simulink library "Wheels_Driver_VehDyn_Lib"  (R2018a)
settings: Solver=VariableStepAuto  StartTime=0.0  StopTime=10.0  RelTol=1e-3
undefined symbols (not defined in the file): I, Kbr, P, vehicleMass
libraries: autolibshared x3, simulink x1
(part 3 of 3)

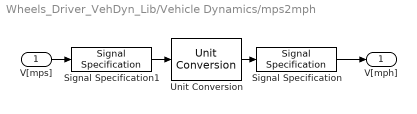
== system Wheels_Driver_VehDyn_Lib/Vehicle Dynamics/mps2mph ==
  V[mps] : Inport
  Signal Specification : SignalSpecification  Unit=mph
  Signal Specification1 : SignalSpecification  Unit=m/s
  Unit Conversion : UnitConversion
  V[mph] : Outport
  wires:
  V[mps]/1 -> Signal Specification1/1
  Unit Conversion/1 -> Signal Specification/1
  Signal Specification1/1 -> Unit Conversion/1
  Signal Specification/1 -> V[mph]/1
